simulink model "inverted_pendulum"  (R2020b)
settings: Solver=FixedStepDiscrete  StartTime=0.0  StopTime=inf  FixedStep=0.002  RelTol=1e-3  EnableMultiTasking=on
values from neighbouring files (symbols this model uses):
  K = lqr(A,B,Q,R)    [inverted_pendulum.m]
  kb = 0.031    [inverted_pendulum.m]
  kt = 0.031    [inverted_pendulum.m]
  r = .006    (= 0.006)    [inverted_pendulum.m]
  Rm = 12.5    [inverted_pendulum.m]
undefined symbols (not defined in the file or in its folder): HIL
libraries: quarc_library x4
settings Model: ExtModeTrigDuration=10000  Creator=student  LastModifiedBy=student
settings SolverCC: PositivePriorityOrder=on
settings DataIOCC: ReturnWorkspaceOutputs=off
settings DebuggingCC: ArithmeticOperatorsInVariantConditions=warning
settings SFSimCC: SimUseLocalCustomCode=off  CustomCodeUndefinedFunction=UseInterfaceOnly
settings RTWCC: Description=QUARC Win64 Target Using Toolchain  SystemTargetFile=quarc_win64.tlc  TemplateMakefile=quarc_default_tmf  RTWUseLocalCustomCode=off  Toolchain=QUARC win64 | nmake (64-bit Windows)  BuildConfiguration=Faster Runs
settings CodeAppCC: StateflowObjectComments=on
settings STFCustomTargetCC: TargetLangStandard=C99 (ISO)  CPPClassGenCompliant=off  UseToolchainInfoCompliant=on
settings GRTTargetCC: ParMdlRefBuildCompliant=off  CompOptLevelCompliant=off  CombineOutputUpdateFcns=off  MatFileLogging=off  CPPClassGenCompliant=off  GRTInterface=on  ExtMode=on  ExtModeMexFile=quarc_comm
settings ConfigComp: CovMetricSettings=dswe

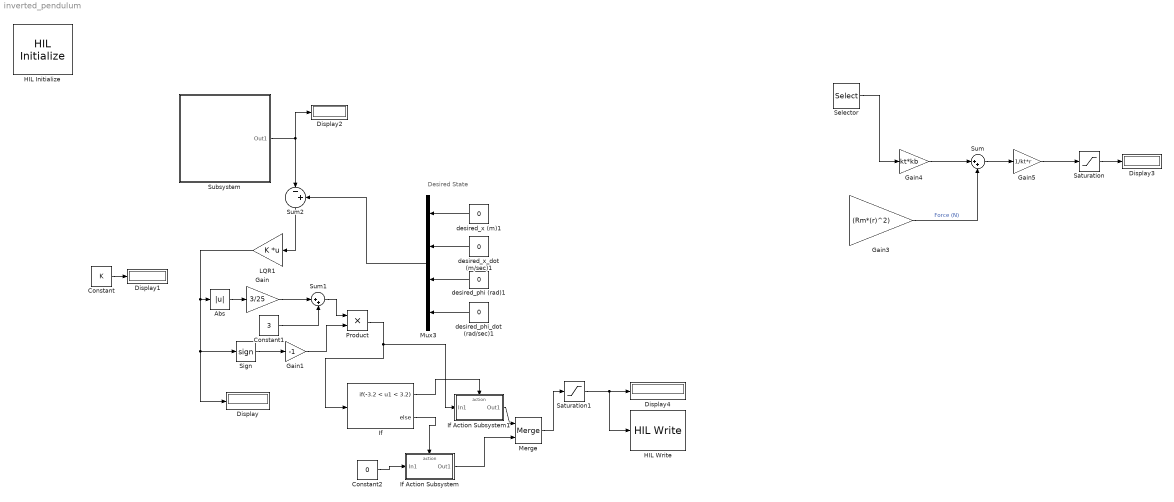
== system inverted_pendulum ==
  note: Desired State
  Abs : Abs
  Constant : Constant  Value=K
  Constant1 : Constant  Value=3
  Constant2 : Constant  Value=0
  Display{,1..4} (5 alike) : Display
      Display4 settings: Decimation=20
  Gain : Gain  Gain=3/25  OutDataTypeStr=double
  Gain1 : Gain  Gain=-1
  Gain3 : Gain  Gain=(Rm*(r)^2)
  Gain4 : Gain  Gain=kt*kb
  Gain5 : Gain  Gain=1/kt*r
  HIL Initialize : quarc_library/Data Acquisition/Generic/Configuration/HIL Initialize  object_name=HIL-1  board_type=q2_usb  board_number=0  board_options=d0=digital;d1=digital;led=auto;update_rate=normal;decimation=1  exclusive=off  active=on  hardware_clocks=[0]  clock_modes=[]  initial_clock_frequencies=[]  set_clock_params_at_start=off  set_clock_params_at_switch_in=off  set_clock_frequencies_at_start=off  set_clock_frequencies_at_switch_in=off  analog_input_channels=[0:1]  analog_input_configurations=[]  analog_input_maximums=10  analog_input_minimums=-10  set_analog_input_params_at_start=on  set_analog_input_params_at_switch_in=off  analog_output_channels=[0:1]  analog_output_maximums=10  analog_output_minimums=-10  initial_analog_outputs=[0]  final_analog_outputs=[0]  watchdog_analog_outputs=0  set_analog_output_params_at_start=on  set_analog_output_params_at_switch_in=off  set_analog_outputs_at_start=on  set_analog_outputs_at_switch_in=off  set_analog_outputs_at_terminate=on  set_analog_outputs_at_switch_out=off  set_analog_outputs_on_watchdog=off  digital_input_channels=[]  digital_output_channels=[]  digital_output_configuration=[]  initial_digital_outputs=[1]  final_digital_outputs=[1]  watchdog_digital_outputs=[1]  set_digital_output_params_at_start=off  set_digital_output_params_at_switch_in=off  set_digital_outputs_at_start=on  set_digital_outputs_at_switch_in=off  set_digital_outputs_at_terminate=on  set_digital_outputs_at_switch_out=off  set_digital_outputs_on_watchdog=off  encoder_channels=[0:1]  quadrature=[4]  encoder_filter_frequency=[]  initial_encoder_counts=[0]  set_encoder_params_at_start=on  set_encoder_params_at_switch_in=off  set_encoder_counts_at_start=on  set_encoder_counts_at_switch_in=off  pwm_channels=[]  pwm_modes=[0]  pwm_frequency=1/0.020  pwm_configuration=[]  pwm_alignment=[]  pwm_polarity=[]  pwm_leading_deadband=[]  pwm_trailing_deadband=[]  initial_pwm_outputs=[0]  final_pwm_outputs=[0]  watchdog_pwm_outputs=[0]  set_pwm_params_at_start=on  set_pwm_params_at_switch_in=off  set_pwm_outputs_at_start=on  set_pwm_outputs_at_switch_in=off  set_pwm_outputs_at_terminate=on  set_pwm_outputs_at_switch_out=off  set_pwm_outputs_on_watchdog=off  other_output_channels=[]  initial_other_outputs=[]  final_other_outputs=[]  watchdog_other_outputs=[]  set_other_outputs_at_start=off  set_other_outputs_at_switch_in=off  set_other_outputs_at_terminate=off  set_other_outputs_at_switch_out=off  set_other_outputs_on_watchdog=off
  HIL Write : quarc_library/Data Acquisition/Generic/Immediate I//O/HIL Write  object_name=HIL-1  analog_channels=1  pwm_channels=[]  digital_channels=[]  other_channels=[]  sample_time=-1  active=off  vector_input=off
  If : If  IfExpression=-3.2 < u1 < 3.2
  If Action Subsystem : Subsystem  TreatAsAtomicUnit=on
  If Action Subsystem1 : Subsystem  TreatAsAtomicUnit=on
  LQR1 : Gain  Gain=K  Multiplication=Matrix(K*u) (u vector)
  Merge : Merge
  Mux3 : Mux
  Product : Product
  Saturation : Saturate  UpperLimit=4  LowerLimit=-4
  Saturation1 : Saturate  UpperLimit=6  LowerLimit=-6
  Selector : Selector  InputPortWidth=4  IndexOptions=Index vector (dialog)  Indices=[2]  OutputSizes=1
  Sign : Signum
  Subsystem : Subsystem
  Sum : Sum  Inputs=|++
  Sum1 : Sum  Inputs=|++
  Sum2 : Sum  Inputs=|-+
  desired_phi (rad)1 : Constant  Value=0
  desired_phi_dot (rad/sec)1 : Constant  Value=0
  desired_x (m)1 : Constant  Value=0
  desired_x_dot (m/sec)1 : Constant  Value=0
  wires:
  Mux3/1 -> Sum2/2
  desired_x (m)1/1 -> Mux3/1
  desired_phi (rad)1/1 -> Mux3/3
  desired_phi_dot (rad/sec)1/1 -> Mux3/4
  desired_x_dot (m/sec)1/1 -> Mux3/2
  Subsystem/1(Out1) -> Sum2/1, Display2/1
  Constant/1 -> Display1/1
  Sum2/1 -> LQR1/1
  Gain3/1 -> Sum/2  "Force (N)"
  Gain4/1 -> Sum/1
  Sum/1 -> Gain5/1
  Selector/1 -> Gain4/1
  Gain5/1 -> Saturation/1
  Saturation/1 -> Display3/1
  Saturation1/1 -> Display4/1, HIL Write/1
  Abs/1 -> Gain/1
  Constant1/1 -> Sum1/2
  Gain/1 -> Sum1/1
  Sum1/1 -> Product/1
  Sign/1 -> Gain1/1
  Gain1/1 -> Product/2
  LQR1/1 -> Display/1, Sign/1, Abs/1
  Product/1 -> If Action Subsystem1/1(In1), If/1
  If/1 -> If Action Subsystem1/Action
  If/2 -> If Action Subsystem/Action
  Constant2/1 -> If Action Subsystem/1(In1)
  If Action Subsystem/1(Out1) -> Merge/2
  If Action Subsystem1/1(Out1) -> Merge/1
  Merge/1 -> Saturation1/1

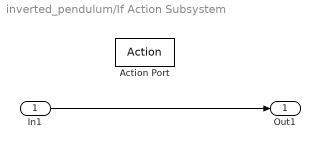
== system inverted_pendulum/If Action Subsystem ==
  In1 : Inport
  Action Port : ActionPort  ActionPortLabel=else
  Out1 : Outport
  wires:
  In1/1 -> Out1/1

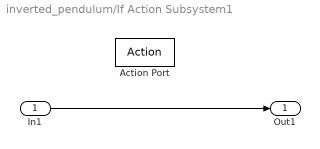
== system inverted_pendulum/If Action Subsystem1 ==
  In1 : Inport
  Action Port : ActionPort  ActionPortLabel=if(-3.2 < u1 < 3.2)
  Out1 : Outport
  wires:
  In1/1 -> Out1/1

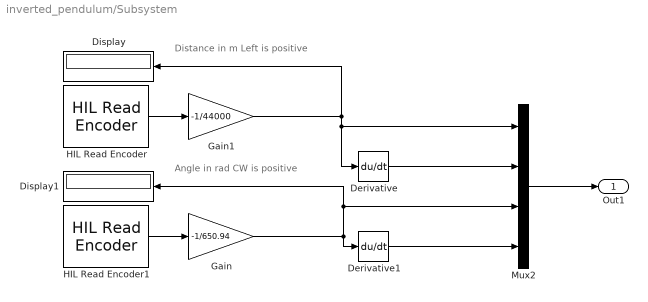
== system inverted_pendulum/Subsystem ==
  note: Distance in m
      | Left is positive
  note: Angle in rad
      | CW is positive
  Derivative : Derivative
  Derivative1 : Derivative
  Display : Display
  Display1 : Display
  Gain : Gain  Gain=-1/650.94
  Gain1 : Gain  Gain=-1/44000
  HIL Read Encoder : quarc_library/Data Acquisition/Generic/Immediate I//O/HIL Read Encoder  object_name=HIL-1  channels=1  sample_time=qc_get_step_size  active=on  vector_output=off  data_type_mode=Inherit via back propagation  data_type=double
  HIL Read Encoder1 : quarc_library/Data Acquisition/Generic/Immediate I//O/HIL Read Encoder  object_name=HIL-1  channels=0  sample_time=qc_get_step_size  active=on  vector_output=off  data_type_mode=Inherit via back propagation  data_type=double
  Mux2 : Mux
  Out1 : Outport
  wires:
  Derivative/1 -> Mux2/2
  Derivative1/1 -> Mux2/4
  Mux2/1 -> Out1/1
  HIL Read Encoder/1 -> Gain1/1
  Gain1/1 -> Mux2/1, Derivative/1, Display/1
  Gain/1 -> Derivative1/1, Display1/1, Mux2/3
  HIL Read Encoder1/1 -> Gain/1
